simulink model "adapt_visodo05_RC"  (Simulink 7.5)
settings: Solver=FixedStepDiscrete  StartTime=0.0  StopTime=100  FixedStep=1  RelTol=1e-3
undefined symbols (not defined in the file): L, R
libraries: simulink x2, vipmorphops x1, vipsnks x1
(part 2 of 2)

== matlab function Adaptation/Adjust Scale or Mask ==
  data: filter_size output double; req_n input double; window input double; Nu input double; res_hist input double; S_tab input double; L_enc input double; num_prev input double; hist_ind output double; f_ind output double; test output double; mean_d_bin input double
function [filter_size,hist_ind,f_ind, test] = decision(req_n,window, Nu, res_hist, S_tab,L_enc, num_prev, mean_d_bin)
% function determines whether to change filter scale or mask size to achieve desired number of matches

persistent c_pers flag_pers f_ind_pers f_mat ef_mat hist_ind_pers
if isempty(f_ind_pers)
    f_ind_pers=4; % start at 2nd largest scale, [38 51 75]
    f_mat=[9 15 21; 15 21 27; 21 27 39; 27 39 51; 39 51 75; 51 75 99];
    hist_ind_pers=1;
    c_pers=0;
    flag_pers=0;
% %     S_mat=[7.5 15.9 24.3 32.7 41.1 49.5]; % feature spacing for each scale (from empirical data)
    ef_mat=[1.5 3.7 4.5 5.4 6 6.5 7 7.7 8.3 8.8 9.3 9.8 10.3 11 11.4 11.8 12.2 12.4 12.9]; 
            % ef for each bin, (from empirical data)
end
S_mat=S_tab;
f_ind=f_ind_pers;
S=S_mat(f_ind); % feature spacing, S, at current scale

beta=.1;
c=c_pers;
flag=flag_pers;
hist_ind=hist_ind_pers;
ipts_bins=res_hist(1,:);
adj_mask=0;
adj_scale=0;
incs_ss=0; % flag for whether higher scale is in sweet spot
decs_ss=0; % flag for whether lower scale is in sweet spot
incz_ss=0;  % flag for whether higher z is in sweet spot
decz_ss=0;  % flag for whether lower z is in sweet spot
c=c+1; 
if num_prev==0 % if no features, jump to histogram bin of mean depth
    hist_ind=mean_d_bin;
    filter_size=f_mat(f_ind,1:3);
    c=0;
    flag=0;
else
    if L_enc==0 % if robot isn't moving (it doesn't look for matches), don't adapt
        c=0; % reset window counter
    elseif c<window  % inside window ==>don't adjust
        flag=flag+req_n; % running sum of hyp. test outcomes
    else % end of window ==>adjust
        flag=flag+req_n;

        % set flags for changing scale
        if f_ind>1
            NuUB_decs=S_mat(f_ind-1)/ef_mat(hist_ind) -1; %Nu upper bound for next lower scale
            if Nu(hist_ind)>(1-beta) && Nu(hist_ind)<(1+beta)*(NuUB_decs)
                decs_ss=1;
            end
        elseif f_ind<6
            NuUB_incs=S_mat(f_ind+1)/ef_mat(hist_ind) -1; %Nu upper bound for next higher scale
            if Nu(hist_ind)>(1-beta) && Nu(hist_ind)<(1+beta)*(NuUB_incs)
                incs_ss=1;
            end
        end
        % set flags for changing mask (z)
        if hist_ind<19
            NuUB_incz=S/ef_mat(hist_ind+1)-1; % Nu upper bound for next range bin
            if Nu(hist_ind+1)>(1-beta) && Nu(hist_ind+1)<(1+beta)*(NuUB_incz)
                incz_ss=1;
            end
        elseif hist_ind>1 && sum(ipts_bins(1:hist_ind-1))>0 % are there ipts in closer bins?
            NuUB_decz=S/ef_mat(hist_ind-1)-1; % Nu upper bound for lower range bin
            if Nu(hist_ind-1)>(1-beta) && Nu(hist_ind-1)<(1+beta)*(NuUB_decz)
                decz_ss=1;
            end
        end

        if flag==0 % sufficient matches in window
            adj_mask=0;
            adj_scale=0;

        elseif flag<0 % not enough matches 
            if decs_ss==1 %
                % decrease scale
                adj_scale=-1;
                adj_mask=0;
            elseif incz_ss==1 %
                % increase mask
                adj_scale=0;
                adj_mask=1;
            else % if neither is in sweet spot
                if f_ind>1 
                    % decrease scale first
                    adj_scale=-1;
                    adj_mask=0;
                elseif hist_ind<19
                    % increase mask
                    adj_scale=0;
                    adj_mask=1;
                end
            end
        elseif flag>0 % too many matches 
            if decz_ss==1
                % decrease mask first (reduce dL)
                adj_scale=0;
                adj_mask=-1;
            elseif incs_ss==1
                % increase scale
                adj_scale=1;
                adj_mask=0;
            else % if neither is in sweet spot
                if hist_ind>1 && sum(ipts_bins(1:hist_ind-1))>5 % are there ipts in closer bins?
                    % decrease mask first
                    adj_scale=0;
                    adj_mask=-1;
                elseif f_ind<6 
                    % increase scale
                    adj_scale=1;
                    adj_mask=0;

                end
            end
        end
        % reset counters
        c=0;
        flag=0;
    end

    % adjust scale logic
    if adj_scale<0 && f_ind>=2
        f_ind=f_ind-1;
    elseif adj_scale>0 && f_ind<=5
        f_ind=f_ind+1;
    end
    filter_size=f_mat(f_ind,1:3);

    % adjust mask logic
    if adj_mask>0
        if hist_ind<19
            hist_ind=hist_ind+1;
        end
    elseif adj_mask<0
        if hist_ind>1
            hist_ind=hist_ind-1;
        end
    end
end % num_prev==0

hist_ind_pers=hist_ind;
f_ind_pers=f_ind;
c_pers=c;
flag_pers=flag;
test=zeros(1,4);
test=[incs_ss decs_ss incz_ss decz_ss];

== matlab function Prev Frame/Epsilon ==
  data: est_ipts input double; eps_vec output double; box input double; num_prev input double; eps output double
function [eps_vec, eps] = calc_eps(est_ipts, box,  num_prev)
% function calculates epsilon for each ipts


%%%%%%%%%%%%%%%%%%%%%%%%%%%%%%%%%%%%%%%%%
%%%%%%%%%%%%%%%%%%%%%%%%%%%%%%%%%%%%%%%%%
% alternate epsilon based on feature closest to z=100cm
eps_vec=zeros(1,1000);
eps=0;
% % if num_prev>0
% %     ave_depth=median(est_ipts(3,1:num_prev));
% %     [val,ind]=min(abs(est_ipts(3,1:num_prev)-ave_depth));
% %     xh=est_ipts(1,ind);
% %     yh=est_ipts(2,ind);
% %     zh=est_ipts(3,ind);
% %     c1x=box(1,ind);
% %     c1z=box(4,ind);
% %     cyt=box(6,ind);
% %     eps=sqrt((c1x-xh)^2+(c1z-zh)^2+(cyt-yh)^2);
% %     
% % end

for n=1:num_prev
    xh=est_ipts(1,n);
    yh=est_ipts(2,n);
    zh=est_ipts(3,n);
    c1x=box(1,n);
    c1z=box(4,n);
    cyt=box(6,n);
    eps_vec(n)=sqrt((c1x-xh)^2+(c1z-zh)^2+(cyt-yh)^2);
end

eps=median(eps_vec(1:num_prev));

== matlab function Matching & Visodo/Feature Matching ==
  data: ipts_rpix input double size=[2 1000]; est_ipts input double; box input double size=[7 1000]; ipts_prev input double; num_prev input double; ipts input double size=[3 1000]; M output double; num_cur input double; num_match output double; miss_count output double; test output double; test2 output double; M_rpix output double
function [M, num_match, miss_count, test,test2, M_rpix] = feat_match(ipts_rpix,est_ipts, box, ipts_prev, num_prev, ipts, num_cur)


persistent miss 
if isempty(miss)
    miss=0; % 
end

max_num_ipts = 1000; %%%%% must be same for 'find_local_extrema', 'uc_to_xk' and 'ipts_to_3Dcolor'

M = zeros(6,max_num_ipts);
M_rpix=uint16(zeros(2,max_num_ipts));
i = 0;
n=0;
same = 0;

% test = uint16(zeros(2,100));
test=zeros(4,1000);
for c = 1:num_cur
    i=i+1;
    index = 0;
    metric = 1000;
    l1=zeros(1,max_num_ipts);
    y=ipts(2,c);
    x=ipts(1,c);
    z=ipts(3,c);
    min_l1=1000;
% %     test2=zeros(4,100);
    for p = 1:num_prev % loop through all est_ipts
        n=n+1;
        l1(1,p) = sum(abs(ipts(:,c)-est_ipts(:,p)));
        same = sum(ipts(:,c)-ipts_prev(:,p)); % =0 if they're the same
        mot = sum(abs(ipts_prev(:,p)-est_ipts(:,p))); % =0 if no motion expected (ie. L=R=0)
% %         test(1,p)=mot;
        xh=est_ipts(1,p);
        left=box(1,p);
        right=box(2,p);
        m=box(3,p);
        z2=box(4,p);
        z4=box(5,p);
        top_y=box(6,p);
        bot_y=box(7,p);
        
        back_z=m*(xh-right)+z2;
        front_z=m*(xh-right)+z4;
% %         test(1,p)=[l1(1,p)];
        
        if mot==0
            index=0; % if no motion (L=R=0) between frames, don't bother checking matches
            break
        elseif x>=left && x<=right && z<=back_z && z>=front_z && y<=top_y && y>=bot_y ...
                 && l1(1,p)<metric && same~=0 
            index = index+1;
            metric = l1(1,p);
            M(1:3,i) = ipts_prev(:,p);
            M(4:6,i) = ipts(:,c); 
            M_rpix(:,i)=ipts_rpix(:,c);
            
        end
        
        if l1(1,p)<min_l1
            min_l1=l1(1,p);
        end
% %         [val,ind]=min(l1(1,1:num_prev));
% %     test(1:4,c)=[val;ind;ipts_rpix(1,ind);ipts_rpix(2,ind)];
    end  % end prev
    test(1:4,c)=[min_l1;double(ipts_rpix(1,c));double(ipts_rpix(2,c));metric];
    if index ==0 % no matches found
        i=i-1; 
    end 
end  % end curr

num_match = i;
% % if num_match==0 % ie, no matches, use est_ipts
% %     miss=miss+1;
% %     M(1:3,1) = ipts_prev(:,1);
% %     M(4:6,1) = est_ipts(:,1);
% % end

miss_count = miss;
% outputs for testing
test2=zeros(6,max_num_ipts);
for p=1:num_prev
    xh=est_ipts(1,p);
    left=box(1,p);
    right=box(2,p);
    m=box(3,p);
    z2=box(4,p);
    z4=box(5,p);
    top_y=box(6,p);
    bot_y=box(7,p);

    back_z=m*(xh-right)+z2;
    front_z=m*(xh-right)+z4;
    test2(:,p)=[left;right;top_y;bot_y;back_z;front_z];
end

== matlab function Model Output ==
  data: time input double; num_cur input double; hist_ind input double; filter input double; matches input double; miss input double; ff_disp input double; cum_disp input double; Sigma input double; Nu input double; mean_d input double; Le input double; output output double; Re input double
%%%%%%%%%%%%%%%%%%%%%%%%
%%%%%%%%%%%%%%%%%%%%%%%%
% code to record 3D displacements of features
function output = model_output(time, num_cur, hist_ind, filter,matches,miss,ff_disp,cum_disp,Sigma,Nu,mean_d,Le,Re)
% generic function to package multiple signals for output to .mat file


output = zeros(25 ,1);
output(1,1) = time;
output(2,1) = num_cur;
output(3,1) = hist_ind;
output(4,1) = filter(2);
output(5,1) = matches;
output(6,1) = miss;
output(13:16,1) = ff_disp(1:4);
output(17:20,1) = cum_disp(1:4);
output(21,1) = Sigma;
output(22,1) = Nu;
output(23,1)= mean_d;
output(24,1)= Le;
output(25,1)= Re;

%%%%%%%%%%%%%%%%%%%%%%%
%%%%%%%%%%%%%%%%%%%%%%%

== matlab function Matching & Visodo/Odometry ==
  data: M input double; ff_disp_av output double; ff_disp_wL output double; cum_disp_av output double; cum_disp_wL output double; num_match input double; L_dist output double; L_vec output double; vo_mean output double; z_wL output double; fr_delay input double; l_hat input double; theta_hat input double
function [ff_disp_av, ff_disp_wL, cum_disp_av, cum_disp_wL,L_dist, L_vec, vo_mean,z_wL] = odometry(M, num_match,fr_delay,l_hat,theta_hat)
% function takes matrix of matches, 'M', and calculates the 
%   - frame-to-frame displacement (straight average and weighted)
%   - cumulative displacement (straight average and weighted)
% Displacement format is: [delta_x 
%                         [delta_z
%                         [l2
%                         [delta_h ]

persistent cum_disp_av_pers cum_disp_wL_pers 
if isempty(cum_disp_av_pers)
    cum_disp_av_pers = [0;0;0;0];
    cum_disp_wL_pers = [0;0;0;0];

end
ff_disp_av = [0;0;0;0];
ff_disp_wL = [0;0;0;0];
vo_mean=[0;0;0;0];
s=0;
L_vec=zeros(1000,1);

n = num_match; 
% % if n==0 %no actual matches, M(:,1)=est_ipts;
% %     n=1;
% % end

ff_disp_vec3 = zeros(4,1000);
z_vec=zeros(1,1000);
cum_disp_av = zeros(4,1);
cum_disp_wL = zeros(4,1);
z_wL = 0;

L_dist=zeros(2,1000);
unc=[0;0];
sL=zeros(1,1000);
sT=zeros(1,1000);
sT2=zeros(1,1000);
disp_av = zeros(4,1);
disp_wL = zeros(4,1);
disp_wT = zeros(4,1);
sum_wL = 0;
sum_wT = 0;

if n==0
    t1=((theta_hat-1.5708)*pi)/2;
    ff_disp_av(1:4,1)=[l_hat*cos(t1) ;l_hat*sin(t1); l_hat; theta_hat];
    ff_disp_wL(1:4,1)=[l_hat*cos(t1) ;l_hat*sin(t1); l_hat; theta_hat];
else
    for i=1:n
        xp = M(1,i); % correct for offset of camera from axle
        zp = M(3,i);
        xc = M(4,i);         
        zc = M(6,i);

        % 3DOF model
        theta1=atan2(zp+zc,xp-xc);
        theta2=theta1-pi;
        theta12=theta1+theta2;
        c12=cos(theta12);
        s12=sin(theta12);
        c1=cos(theta1);
        s1=sin(theta1);
% %         L3=(xp-c12*xc+s12*zc)/c1;
        L3=(zp-s12*xc-c12*zc)/s1;
        delta_x3=L3*cos(theta1);
        delta_z3=L3*sin(theta1);
        ff_disp_vec3(1:4,i)=[delta_x3;delta_z3;L3;theta12];
        z_vec(i)=zc;
        
        % calculate uncertainties for weighting average solution
        sxp2=2e-4*xp^2;
        sxc2=2e-4*xc^2;
        szp2=2e-10*zp^4;
        szc2=2e-10*zc^4;
% %         sT(1,i)=(1.4142*abs(xp-xc)/((xp-xc)^2+(zp+zc)^2))*sqrt(szp2+szc2+tan(theta1)^2*(sxp2+sxc2)) + 1e-10;  %% 1e-10 added to avoid singularlity in weighted average sL(1,i)=abs(1/s1)*sqrt(szp2+s12^2*sxc2+c12^2*szc2+(-c12*xc+s12*zc)^2*sT(1,i)^2+c1^2*L3^2*(sT(1,i)/1.4142)^2);
        sL(1,i)=abs(1/s1)*sqrt(szp2+s12^2*sxc2+c12^2*szc2+(-c12*xc+s12*zc)^2*sT(1,i)^2+c1^2*L3^2*(sT(1,i)/1.4142)^2);
        L_dist(1:2,i)=[L3/(fr_delay+1);zc];      
        L_vec(i,1)=L3;
% %         t_vec(i,1)=theta12;
    end % i

    s=std(ff_disp_vec3(3,1:n));
    vo_mean=mean(ff_disp_vec3(:,1:n),2);

    if n>1
        sL_max=max(sL(1:n));
        sL_min=min(sL(1:n));

        for i=1:n
            wL=(sL(i).^-1-sL_max.^-1)./(sL_min.^-1-sL_max.^-1);
            if isnan(wL)
                wL=0;
            end
            disp_av=ff_disp_vec3(1:4,i) + disp_av;
            disp_wL=wL.*ff_disp_vec3(1:4,i) + disp_wL;
            z_wL=wL*z_vec(i)+z_wL;
            sum_wL=sum_wL+wL;
        end
            ff_disp_av = disp_av./n;
            ff_disp_wL = disp_wL./sum_wL;
            z_wL=z_wL/sum_wL;
    else
        ff_disp_av=ff_disp_vec3(:,1);
        ff_disp_wL=ff_disp_vec3(:,1);
    end


    if isnan(ff_disp_av(1,1))
        ff_disp_av = [0;0;0;0];
    end
    if isnan(ff_disp_wL(1,1))
        ff_disp_wL = [0;0;0;0];
    end

    % average over skipped frames
    ff_disp_av=ff_disp_av./(fr_delay+1);
    ff_disp_wL=ff_disp_wL./(fr_delay+1);
end

% calculate cumulative visodo
%% based on straight average...
cum_disp_av(3,1) = cum_disp_av_pers(3,1) + ff_disp_av(3,1); % L
cum_disp_av(4,1) = cum_disp_av_pers(4,1) + ff_disp_av(4,1); % dh
cum_disp_av(1,1)=cum_disp_av_pers(1,1) - (ff_disp_av(3,1))*sin(cum_disp_av_pers(4,1)+(ff_disp_av(4,1))/2); % cum x
cum_disp_av(2,1)=cum_disp_av_pers(2,1) + (ff_disp_av(3,1))*cos(cum_disp_av_pers(4,1)+(ff_disp_av(4,1))/2); % cum z

%% weighted by uncertainty in L...
cum_disp_wL(3,1) = cum_disp_wL_pers(3,1) + ff_disp_wL(3,1); % L
cum_disp_wL(4,1) = cum_disp_wL_pers(4,1) + ff_disp_wL(4,1); % dh
cum_disp_wL(1,1)=cum_disp_wL_pers(1,1) - (ff_disp_wL(3,1))*sin(cum_disp_wL_pers(4,1)+(ff_disp_wL(4,1))/2); % cum x
cum_disp_wL(2,1)=cum_disp_wL_pers(2,1) + (ff_disp_wL(3,1))*cos(cum_disp_wL_pers(4,1)+(ff_disp_wL(4,1))/2); % cum z

% store persistent variables
cum_disp_av_pers = cum_disp_av;
cum_disp_wL_pers = cum_disp_wL;

== matlab function Adaptation/Depth Mask ==
  data: hist_ind input double; mask_im_pad output double; mask_pts output double; hist input double; bins input double; d_cm input double; num_mask output double; max_d output double
function [mask_im_pad,mask_pts, num_mask,max_d] = make_mask(hist_ind, hist, bins, d_cm)
% function analyzes depth histgram and creates mask of nearest pixels...converted (approx) to RGB space

h=size(d_cm,1);
w=size(d_cm,2);
mask_pts=zeros(3,44800);
mask_im_pad=zeros(h,w);
thresh=uint16(0);
max_d_ind=hist_ind;
pad=4;

d_hist=hist(1,:);

% build mask of depth image
thresh=bins(2,max_d_ind);
max_d=thresh;
count=0;
vert_offset=10;
for dj=1:h-vert_offset % index in depth
    j=dj+vert_offset; % index in registered mask
    for di=7:w
        i=di+round(-0.08*di+7);
        if d_cm(dj,di)<=thresh && d_cm(dj,di)>0;
            count=count+1;
            mask_pts(1:3,count)=[j;i;d_cm(dj,di)];
            mask_im_pad(j,i)=d_cm(dj,di);
            % pad mask as function scans right then down
            if dj>pad && di>pad && mask_im_pad(j,i-1)==0% edge pixel in mask, going right
                for p=1:pad
                    if d_cm(dj,di-p)<1000;
                        count=count+1;
                        mask_pts(1:3,count)=[j;i-p;d_cm(dj,di-p)];
                        mask_im_pad(j,i-p)=d_cm(dj,di-p);
                    end
                end
            end
            if dj>pad && di>pad && mask_im_pad(j-1,i)==0% edge pixel in mask, going down
                for p=1:pad
                    if d_cm(dj-p,di)<1000;
                        count=count+1;
                        mask_pts(1:3,count)=[j-p;i;d_cm(dj-p,di)];
                        mask_im_pad(j-p,i)=d_cm(dj-p,di);
                    end
                end
            end
        elseif di>1 && d_cm(dj,di)>thresh && d_cm(dj,di-1)<=thresh % right edge in mask, going right
            for p=0:pad-1
                if di<w-p && d_cm(dj,di+p)<1000 
                    count=count+1;
                    mask_pts(1:3,count)=[j;i+p;d_cm(dj,di+p)];
                    mask_im_pad(j,i+p)=d_cm(dj,di+p);
                end
            end
        elseif dj>1 && d_cm(dj,di)>thresh && d_cm(dj-1,di)<=thresh % bottom edge in mask, going down
            for p=0:pad-1
                if dj<h-p && d_cm(dj+p,di)<1000 
                    count=count+1;
                    mask_pts(1:3,count)=[j+p;i;d_cm(dj+p,di)];
                    mask_im_pad(j,i+p)=d_cm(dj+p,di);
                end
            end
        end
        
    end
end
num_mask=count;

== matlab function Adaptation/Compute Stats ==
  data: num_match_prev input double; res_hist input double size=[8,19]; Ln output double; sn output double; bins input double; Nu output double; Sigma output double; SEM output double; ef output double; max_d_ind input double; Nu_av output double; Sigma_av output double
function [Ln, sn, Nu,Sigma, SEM,ef, Nu_av,Sigma_av] = stats(num_match_prev,res_hist, bins, max_d_ind)
% function computes relevant stats from res_hist

persistent z_pers
if isempty(z_pers)
    z_pers=zeros(2,19);
    z_pers(:,1)=[50; 125];
    for i=2:19
        z_pers(1,i)=z_pers(2,i-1); % front of bin
        z_pers(2,i)=sqrt(13125+z_pers(1,i)^2); % back of bin
    end
end
if isempty(res_hist) % initialize for first frame
    res_hist=zeros(8,19);
end

% calculate weighted average and stddev depth
ef=0;
w=zeros(1,19);
match=res_hist(6,1:19);
for m=1:19
    if match(m)~=0
        w(m)=match(m)./num_match_prev;
    else
        w(m)=0;
    end
end
mean_d=sum(bins(2,1:19).*w(1,1:19)); 
Ln=sum(res_hist(7,1:19).*w(1,1:19)); % weighted average of L, per bin
sn=sum(res_hist(8,1:19).*w(1,1:19)); % weighted stddev of L, per bin
Nu_w_temp=0;
Sigma_w_temp=0;
c=0;
for b=1:19
    if w(b)~=0
        c=c+1;
        Nu_w_temp=Nu_w_temp+(res_hist(5,b)./res_hist(4,b)); % weighted ave of Nu, per bin
        Sigma_w_temp=Sigma_w_temp+(res_hist(3,b)./(2.*res_hist(4,b))); % weighted ave of Sigma, per bin
    end
end
Nu_av=Nu_w_temp/c;
Sigma_av=Sigma_w_temp/c;

SEbin=res_hist(8,:)./sqrt(res_hist(6,:));
for i=1:19
    if isnan(SEbin(i))
        SEbin(i)=0;
    end
end
SEM=sum(SEbin.*w(1,1:19)); % weighted stddev of L, per bin
% find bin with most features
% % [val, ind]=max(res_hist(1,:));
% % most=ind;

% calculate Nu and Nu_UB for last bin in mask
Nu=zeros(1,19);
% % Nu_UB=zeros(1,3);
Nu=res_hist(5,:)./res_hist(4,:); % eps/ef
% % SEM=res_hist(8,:)./sqrt(res_hist(6,:));  % sn/sqrt(n)
ef=res_hist(4,max_d_ind);
S=res_hist(3,max_d_ind);
Sigma=S/(2*ef); % Sigma=S/2ef

== matlab function Prev Frame/ipts spacing ==
  data: num_prev input double; ipts_prev input double; S output double; S_mean output double
function [S,S_mean]  = spacing(num_prev, ipts_prev)
% function calculates distance to nearest ipts for each ipts in a single frame

persistent min_spacing_pers
if isempty(min_spacing_pers)
    min_spacing_pers=0;
end

ipts = ipts_prev;
dist = zeros(1,999)+1000;
min_dist = zeros(1,1000)+1000;
S=zeros(1,1000);

for i=1:num_prev
    index = 0;
    if ipts(1,i)~=0
        for j=1:num_prev
            if j~=i && ipts(1,j)~=0
                index=index+1;
                dist(index) = sqrt((ipts(1,i)-ipts(1,j))^2 + (ipts(2,i)-ipts(2,j))^2 + (ipts(3,i)-ipts(3,j))^2);
            end
        end % j
    end
    min_dist(i) = min(dist); % closest neighbor for each ipts  

    if num_prev < 2
        min_dist(i)=min_spacing_pers(1,1);
    end
end % i

% % space = min(min_dist);
% % if space<min_spacing
% %     min_spacing=space
% % end
% % space=min_spacing;

% compute median of nearest neighbors
S(1:num_prev) = (min_dist(1:num_prev));%std(min_dist(1:num_cur))];
S_mean=mean(S(1:num_prev));
min_spacing_pers(1) = S(1,1);
